simulink model "untitled1"  (R2025a)
settings: Solver=VariableStepAuto  StartTime=0.0  StopTime=36  MaxStep=1e-4  RelTol=1e-3
values from neighbouring files (symbols this model uses):
  alpha = 50    [Planning_Adaptive_LTV.m]
  beta = 5    [Planning_Adaptive_LTV.m]
  gamma = 10    [Planning_Adaptive_LTV.m]
  initial_positions_rad = rawJointPositions(1, :)'    [manipulator_sim.m]
  N = numel(theta_points_rad)    [create_LPV_linearizer.m]
  waypoints = pathObj.States(:, 1:2)    [Planning_Adaptive_LTV.m]
  x0 = zeros(10, 1)    [Planning_Adaptive_LTV.m]
undefined symbols (not defined in the file or in its folder): p, X, Y, Z
libraries: sm_lib x181, nesl_utility x29, fl_lib x3, simulink x2, eeGeneralControl x1
(part 5 of 5)

== matlab function untitled1/MATLAB Function7 ==
  settings: updateMethod=DISCRETE
  data: x input; phi_dot_c output; p parameter; simtime input; waypoints input
function phi_dot_c  = generate_ff_fb_velocity_command(x, p, simtime, waypoints)
% =========================================================================
% ADVANCED FEEDFORWARD + FEEDBACK VELOCITY COMMAND GENERATOR
%
% Version: 5.0 - Hybrid Control for Final Approach
%
% This version uses the advanced path-following controller for the main
% trajectory and switches to a simple proportional position controller
% for the final segment to ensure stable regulation at the goal.
% =========================================================================

% --- Parametri ---
persistent processed_path;
persistent previous_waypoints;
v_max       = 0.4;
a_max       = 0.1;
Kp_feedback = 0.3; % Gain for path following on intermediate segments
lookahead_distance = 0.3;

% NEW: Proportional gain specifically for the final approach/regulation.
% You can tune this gain to get the desired stopping behavior.
Kp_final_approach = 1;

% --- Stato attuale del robot ---
p_current = [p.r_S * x(7); -p.r_S * x(3)];
v_current = [p.r_S * x(8); -p.r_S * x(4)];

% --- Logica di Inizializzazione e Replanning (invariata) ---
if isempty(previous_waypoints)
    disp('First run: Initializing and processing path...');
    processed_path = preprocess_waypoints_with_blending(waypoints, v_max, a_max, ...
                                                        p_current, v_current, simtime);
    previous_waypoints = waypoints;
else
    if ~isequal(waypoints, previous_waypoints)
        disp('Waypoints changed: Replanning path from current state...');
        processed_path = preprocess_waypoints_with_blending(waypoints, v_max, a_max, ...
                                                            p_current, v_current, simtime);
        previous_waypoints = waypoints;
    end
end

% --- MODIFIED: HYBRID CONTROL LOGIC ---

% Get the current trajectory information, including the segment index
[v_ref_normal, current_segment, segment_is_valid, current_segment_idx] = get_reference_and_segment(processed_path, simtime);
num_total_segments = length(processed_path.segments);

% Check if we are on the final segment of the path.
is_final_segment = (segment_is_valid && current_segment_idx == num_total_segments);

if is_final_segment
    % --- FINAL APPROACH: Simple Proportional Regulation Controller ---
    %disp('Final segment: Using regulation controller.');
    
    p_goal = waypoints(end, :)'; % The final destination
    position_error = p_goal - p_current;
    
    % The velocity command is purely proportional to the position error.
    v_cmd = Kp_final_approach * position_error;
    
else
    % --- PATH FOLLOWING: Advanced Controller for Intermediate Segments ---
    
    % This is the original advanced logic
    if segment_is_valid
        vec_start_to_robot = p_current - current_segment.p_start;
        projection_dist = dot(vec_start_to_robot, current_segment.direction);
        p_closest = current_segment.p_start + projection_dist * current_segment.direction;
        p_lookahead = p_closest + lookahead_distance * current_segment.direction;
        vec_start_to_lookahead = p_lookahead - current_segment.p_start;
        dist_start_to_lookahead = dot(vec_start_to_lookahead, current_segment.direction);
        if dist_start_to_lookahead > current_segment.distance
            p_target_for_feedback = current_segment.p_end;
        else
            p_target_for_feedback = p_lookahead;
        end
    else
        p_target_for_feedback = p_current; 
    end
    
    position_error = p_target_for_feedback - p_current;
    v_feedback = Kp_feedback * position_error;
    
    % Combine feedforward (from trapezoidal profile) and feedback
    v_cmd = v_ref_normal + v_feedback;
end

% --- Override for initialization phase (remains the same) ---
initialization_time = 3.0;
if simtime < initialization_time
    position_error_init = [0;0] - p_current;
    v_cmd = Kp_final_approach * position_error_init; % Use the regulation controller to hold at zero
end

% --- Final command generation (acts on v_cmd from either logic branch) ---
v_cmd_magnitude = norm(v_cmd);
if v_cmd_magnitude > v_max
    v_cmd = v_cmd / v_cmd_magnitude * v_max;
end
phi_dot_c = [v_cmd(1) / p.r_S; -v_cmd(2) / p.r_S];

end

% =========================================================================
% --- LOCAL HELPER FUNCTIONS ---
% =========================================================================
function processed_path = preprocess_waypoints_with_blending(waypoints, v_max, a_max, p_start_robot, v_start_robot, time_start_robot)
    
    effective_waypoints = [p_start_robot'; waypoints']
    num_waypoints = size(effective_waypoints, 1);
    num_segments = num_waypoints - 1;
    
    % --- Calcolo della geometria (invariato) ---
    segment_template = struct('p_start', zeros(2,1), 'p_end', zeros(2,1), 'distance', 0, 'direction', zeros(2,1));
    path_geom.segments = repmat(segment_template, 1, num_segments);
    for i = 1:num_segments
        p_start = effective_waypoints(i, :)';
        p_end   = effective_waypoints(i+1, :)';
        vec     = p_end - p_start;
        dist    = norm(vec);
        path_geom.segments(i).p_start   = p_start;
        path_geom.segments(i).p_end     = p_end;
        path_geom.segments(i).distance  = dist;
        if dist > 1e-6
            path_geom.segments(i).direction = vec / dist;
        else
            path_geom.segments(i).direction = zeros(2,1);
        end
    end
    
    % --- Calcolo delle velocità di transizione ---
    v_transitions = zeros(2, num_waypoints);
    v_transitions(:, 1) = v_start_robot;
    v_transitions(:, end) = [0; 0];
    alpha = 1.0;
    
    % MODIFIED: Corrected loop range to include the penultimate waypoint
    for i = 2:num_waypoints-1
        v_max_for_corner = v_max;
        % MODIFIED: Slow down for the corners leading into the last TWO segments
        if i >= num_waypoints - 2 
            v_max_for_corner = v_max / 2;
        end
        
        dir_in  = path_geom.segments(i-1).direction;
        dir_out = path_geom.segments(i).direction;
        cos_theta = dot(dir_in, dir_out);
        v_mag = v_max_for_corner * ((1 + cos_theta) / 2)^alpha;
        v_dir_vec = dir_in + dir_out;
        if norm(v_dir_vec) > 1e-6
            v_dir_normalized = v_dir_vec / norm(v_dir_vec);
        else
            v_dir_normalized = zeros(2,1);
            v_mag = 0;
        end
        v_transitions(:, i) = v_mag * v_dir_normalized;
    end
    
    % --- Calcolo del profilo trapezoidale per ogni segmento ---
    profile_template = struct('v_start',0,'v_cruise',0,'v_end',0,'t_accel',0,'t_const',0,'t_decel',0,'total_time',0,'start_time',0,'a_max',0);
    processed_segment_template = struct('profile',profile_template,'direction',zeros(2,1),'p_start',zeros(2,1),'p_end',zeros(2,1),'distance',0);
    processed_segments = repmat(processed_segment_template, 1, num_segments);
    
    cumulative_time = time_start_robot;
    for i = 1:num_segments
        % MODIFIED: Set v_max and a_max for the last TWO segments
        v_max_current = v_max;
        a_max_current = a_max;
        if i >= num_segments - 1 && num_segments > 1 % Check if it's one of the last two segments
            v_max_current = v_max / 2;
            a_max_current = a_max / 2;
        elseif num_segments == 1 % Handle the case of a single-segment path
             v_max_current = v_max / 2;
             a_max_current = a_max / 2;
        end

        segment = path_geom.segments(i);
        v_start = dot(v_transitions(:, i),   segment.direction);
        v_end   = dot(v_transitions(:, i+1), segment.direction);
        v_start = max(0, v_start);
        v_end   = max(0, v_end);
        
        dist_accel = (v_max_current^2 - v_start^2) / (2 * a_max_current);
        dist_decel = (v_max_current^2 - v_end^2)   / (2 * a_max_current);

        if (dist_accel + dist_decel) >= segment.distance
            v_peak_sq = (2*a_max_current*segment.distance + v_start^2 + v_end^2) / 2;
            v_cruise = sqrt(max(0, v_peak_sq));
            t_accel = (v_cruise - v_start) / a_max_current;
            t_const = 0;
            t_decel = (v_cruise - v_end) / a_max_current;
        else
            v_cruise = v_max_current;
            dist_const = segment.distance - dist_accel - dist_decel;
            t_accel = (v_cruise - v_start) / a_max_current;
            t_const = dist_const / v_cruise;
            t_decel = (v_cruise - v_end) / a_max_current;
        end
        
        processed_segments(i).profile.v_start  = v_start;
        processed_segments(i).profile.v_cruise = v_cruise;
        processed_segments(i).profile.v_end    = v_end;
        processed_segments(i).profile.t_accel  = max(0, t_accel);
        processed_segments(i).profile.t_const  = max(0, t_const);
        processed_segments(i).profile.t_decel  = max(0, t_decel);
        processed_segments(i).profile.total_time = processed_segments(i).profile.t_accel + processed_segments(i).profile.t_const + processed_segments(i).profile.t_decel;
        processed_segments(i).profile.start_time = cumulative_time;
        processed_segments(i).profile.a_max = a_max_current;
        
        processed_segments(i).direction = segment.direction;
        processed_segments(i).p_start = segment.p_start;
        processed_segments(i).p_end = segment.p_end;
        processed_segments(i).distance = segment.distance;
        
        cumulative_time = cumulative_time + processed_segments(i).profile.total_time;
    end
    processed_path.segments = processed_segments;
    processed_path.total_duration = cumulative_time;
end
% MODIFIED: Returns a fixed-size struct and a validity flag.
function [v_ref, segment, is_valid, current_segment_idx] = get_reference_and_segment(processed_path, simtime)
    % 1. Define templates
    profile_template = struct(...
        'v_start', 0, 'v_cruise', 0, 'v_end', 0, ...
        't_accel', 0, 't_const', 0, 't_decel', 0, ...
        'total_time', 0, 'start_time', 0, 'a_max', 0);
        
    segment_template = struct(...
        'profile', profile_template, 'direction', zeros(2,1), ...
        'p_start', zeros(2,1), 'p_end', zeros(2,1), 'distance', 0);
    
    % 2. Initialize outputs
    segment = segment_template; 
    v_ref = [0;0];
    is_valid = false;
    
    % FIX: Initialize the new output variable to a default value.
    % This ensures it is always defined, even if the 'if' block is skipped.
    current_segment_idx = 0; 
    
    % 3. Main Logic (This part is unchanged and correct)
    if ~isempty(processed_path) && ~isempty(processed_path.segments)
        % This loop finds the correct segment index and overwrites the default '0'
        for i = 1:length(processed_path.segments)
            if simtime >= processed_path.segments(i).profile.start_time
                current_segment_idx = i;
            else
                break;
            end
        end
        segment = processed_path.segments(current_segment_idx);
        is_valid = true;
        prof = segment.profile;
        
        a_max_current = prof.a_max; 
        
        if simtime >= processed_path.total_duration
            v_ref = [0; 0];
            return;
        end
        time_in_segment = simtime - prof.start_time;
        current_speed = 0.0;
        
        if time_in_segment < prof.t_accel
            current_speed = prof.v_start + a_max_current * time_in_segment;
        elseif time_in_segment < (prof.t_accel + prof.t_const)
            current_speed = prof.v_cruise;
        else
            time_in_decel = time_in_segment - (prof.t_accel + prof.t_const);
            current_speed = prof.v_cruise - a_max_current * time_in_decel;
        end
        v_ref = max(0, current_speed) * segment.direction;
    end
end

== matlab function untitled1/MATLAB Function ==
  data: x_m input; r input; theta_EQ input; dx_m output
function dx_m = saggital_model(x_m, r, theta_EQ)

Am_x = saggital_Am_func(theta_EQ);
Bm_x = saggital_Bm_func(theta_EQ);

A_norm = norm(Am_x);
B_norm = norm(Bm_x);
dx_m = Am_x * x_m + Bm_x * r;

== matlab function untitled1/Subsystem/MATLAB Function4 ==
  data: ye_x output; ye_r output; e input; ye output; x input; r input
function [ye_x, ye_r,ye] = y_e_computation(e, x, r)
B = roll_B_func(x(1));
P = saggital_Pm_func(x(1));
ye = B'*P*e;
ye_x = ye*x';
ye_r = ye*r';

== matlab function untitled1/Subsystem/MATLAB Function2 ==
  data: r input; K input; Kr input; KE input; u output; x input; ye_sw_act input
function u = controller(r, K,Kr,KE,x,ye_sw_act)
u = K*x+Kr*r+KE*ye_sw_act;

== matlab function untitled1/Subsystem/MATLAB Function3 ==
  data: KE output; Kr output; yex input; K output; int_yex input; yer input; int_yer input; int_ye_abs input; alpha parameter; beta parameter; gamma parameter
function [KE, Kr, K] = adapt_law(yex, int_yex, yer, int_yer, int_ye_abs, alpha, beta, gamma)
     
    K= alpha* int_yex + beta*yex;
    Kr= alpha * int_yer + beta*yer;
    KE = gamma * int_ye_abs;

end

== matlab function untitled1/MATLAB Function1 ==
  data: x_m input; r input; theta_EQ input; dx_m output
function dx_m = frontal_model(x_m, r, theta_EQ)

Am_x = frontal_Am_func(theta_EQ);
Bm_x = frontal_Bm_func(theta_EQ);

A_norm = norm(Am_x);
B_norm = norm(Bm_x);

dx_m = Am_x * x_m + Bm_x * r;

== matlab function untitled1/MATLAB Function3 ==
  data: x_m input; r input; dx_m output
function dx_m = yaw_model(x_m, r)

Am_z = yaw_Am_func(r);
Bm_z = yaw_Bm_func(r);

dx_m = Am_z * x_m + Bm_z * r;

== matlab function untitled1/MATLAB Function4 ==
  data: x input; p parameter; wrench_ext input; tau input; dx output
function dx = stateDerivative3D_with_exforce(x, p, wrench_ext,tau)
    % MODIFICATION 1: The function now accepts a 4th argument, 'wrench_ext',
    % which is a vector containing the external forces and torques from Simulink.


    % Unpack state vector (10 elements)
    theta_x = x(1); 
    dot_theta_x = x(2);
    % phi_x = x(3); % Not needed for dynamicsù
    dot_phi_x   = x(4);

    theta_y = x(5); 
    dot_theta_y = x(6);
    % phi_y   = x(7); % Not needed for dynamics
    dot_phi_y   = x(8);

    theta_z = x(9); 
    dot_theta_z = x(10);

    % Unpack input torques
    tau_x = tau(1);
    tau_y = tau(2);
    tau_z = tau(3);

     % Unpack the external wrench vector from the new input ---
    % Expected order: [F_px, F_py, F_pz, tau_px, tau_py]
    F_px   = wrench_ext(1);
    F_py   = wrench_ext(2);
    F_pz   = wrench_ext(3);
    tau_px = wrench_ext(4);
    tau_py = wrench_ext(5);
    tau_pz = wrench_ext(6);

    % --- Prepare arguments for auto-generated functions ---
    % Create separate parameter vectors for each plane, now including h_app
    % Note: I_Ux is for roll, I_Uy is for pitch.
    params_arg_roll = [p.m_U, p.I_Uy, p.I_Ux, p.l_U, p.m_S, p.I_S, p.r_S, p.g, p.b_theta, p.b_phi, p.h_app];
    params_arg_pitch = [p.m_U,p.I_Uy, p.I_Ux, p.l_U, p.m_S, p.I_S, p.r_S, p.g, p.b_theta, p.b_phi, p.h_app];

    external_vars_x = [F_py, F_pz, tau_px]; % For Roll dynamics
    external_vars_y = [F_px, F_pz, tau_py]; % For Pitch dynamics

    % --- X-Z Plane (Roll) Dynamics ---
    states_arg_x = [theta_x, dot_theta_x, dot_phi_x];
    inputs_arg_x = [tau_x];
    ddot_theta_x = copy_autogen_ddot_theta_x(states_arg_x, inputs_arg_x, params_arg_roll,external_vars_x);
    ddot_phi_x   = copy_autogen_ddot_phi_x(states_arg_x, inputs_arg_x, params_arg_roll,external_vars_x);


    % --- Y-Z Plane (Pitch) Dynamics ---
    states_arg_y = [theta_y, dot_theta_y, dot_phi_y];
    inputs_arg_y = [tau_y];
    ddot_theta_y = copy_autogen_ddot_theta_y(states_arg_y, inputs_arg_y, params_arg_pitch,external_vars_y);
    ddot_phi_y   = copy_autogen_ddot_phi_y(states_arg_y, inputs_arg_y, params_arg_pitch,external_vars_y);

    % --- Transversal Plane Dynamics (Yaw) ---
    % external forces at the center of the top surface are assumed not to produce yaw torque.
    ddot_theta_z = (tau_z + tau_pz- p.fz * dot_theta_z) / p.Iz;

    % --- Assemble the state derivative vector dx ---
    dx = [
        dot_theta_x;    % dx(1) = d(theta_x)/dt
        ddot_theta_x;   % dx(2) = d(dot_theta_x)/dt
        dot_phi_x;      % dx(3) = d(phi_x)/dt
        ddot_phi_x;     % dx(4) = d(dot_phi_x)/dt

        dot_theta_y;    % dx(5) = d(theta_y)/dt 
        ddot_theta_y;   % dx(6) = d(dot_theta_y)/dt
        dot_phi_y;      % dx(7) = d(phi_y)/dt
        ddot_phi_y;     % dx(8)= d(dot_phi_y)/dt

        dot_theta_z;    % dx(9) = d(theta_z)/dt
        ddot_theta_z;   % dx(10) = d(dot_theta_z)/dt
    ];
end

% function dx = stateDerivative3D_generated(x, tau, p)
%     % SW was assumed to not spin relative to the ground
% 
%     % Unpack state vector (10 elements)
%     theta_x = x(1); 
%     dot_theta_x = x(2);
%     % phi_x = x(3); % Not needed for dynamicsù
%     dot_phi_x   = x(4);
% 
%     theta_y = x(5); 
%     dot_theta_y = x(6);
%     % phi_y   = x(7); % Not needed for dynamics
%     dot_phi_y   = x(8);
% 
%     theta_z = x(9); 
%     dot_theta_z = x(10);
% 
%     % Unpack input torques
%     tau_x = tau(1);
%     tau_y = tau(2);
%     tau_z = tau(3);
% 
%     % --- Prepare arguments for auto-generated functions ---
%     % Argument list for parameters (order MUST match the generator script)
%     params_arg = [p.m_U, p.I_Uy, p.I_Ux, p.l_U, p.m_S, p.I_S, p.r_S, p.g, p.b_theta, p.b_phi];
% 
%     % --- X-Z Plane (Roll) Dynamics ---
%     states_arg_x = [theta_x, dot_theta_x, dot_phi_x];
%     inputs_arg_x = [tau_x];
%     ddot_theta_x = autogen_ddot_theta_x(states_arg_x, inputs_arg_x, params_arg);
%     ddot_phi_x   = autogen_ddot_phi_x(states_arg_x, inputs_arg_x, params_arg);
% 
%     % --- Y-Z Plane (Pitch) Dynamics ---
%     states_arg_y = [theta_y, dot_theta_y, dot_phi_y];
%     inputs_arg_y = [tau_y];
%     ddot_theta_y = autogen_ddot_theta_y(states_arg_y, inputs_arg_y, params_arg);
%     ddot_phi_y   = autogen_ddot_phi_y(states_arg_y, inputs_arg_y, params_arg);
% 
%     % --- Transversal Plane Dynamics (Yaw) ---
%     % Using the simple decoupled model from your original script
%     ddot_theta_z = (tau_z - p.fz * dot_theta_z) / p.Iz;
% 
%     % --- Assemble the state derivative vector dx ---
%     dx = [
%         dot_theta_x;    % dx(1) = d(theta_x)/dt
%         ddot_theta_x;   % dx(2) = d(dot_theta_x)/dt
%         dot_phi_x;      % dx(3) = d(phi_x)/dt
%         ddot_phi_x;     % dx(4) = d(dot_phi_x)/dt
% 
%         dot_theta_y;    % dx(5) = d(theta_y)/dt 
%         ddot_theta_y;   % dx(6) = d(dot_theta_y)/dt
%         dot_phi_y;      % dx(7) = d(phi_y)/dt
%         ddot_phi_y;     % dx(8)= d(dot_phi_y)/dt
% 
%         dot_theta_z;    % dx(9) = d(theta_z)/dt
%         ddot_theta_z;   % dx(10) = d(dot_theta_z)/dt
%     ];
% end
